simulink model "QAM"  (R2021b)
settings: Solver=VariableStepAuto  StartTime=0.0  StopTime=10.0  RelTol=1e-3
undefined symbols (not defined in the file or in its folder): magnitude
libraries: dspxfrm3 x3, dspsigops x3, commdigbbndam3 x2, commchan3 x1, commrandsrc3 x1
settings Model: Creator=malth  LastModifiedBy=malth

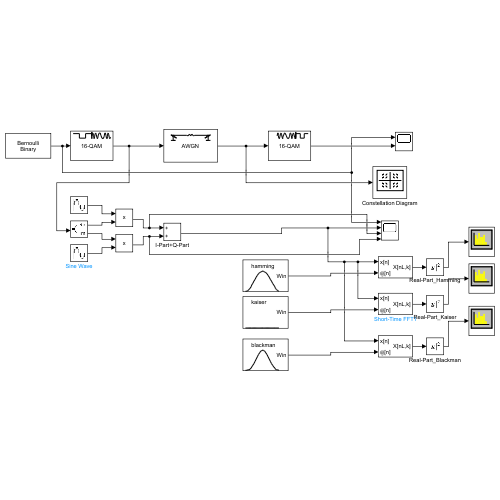
[thumbnail: Simulink's stored preview of the top-level diagram]
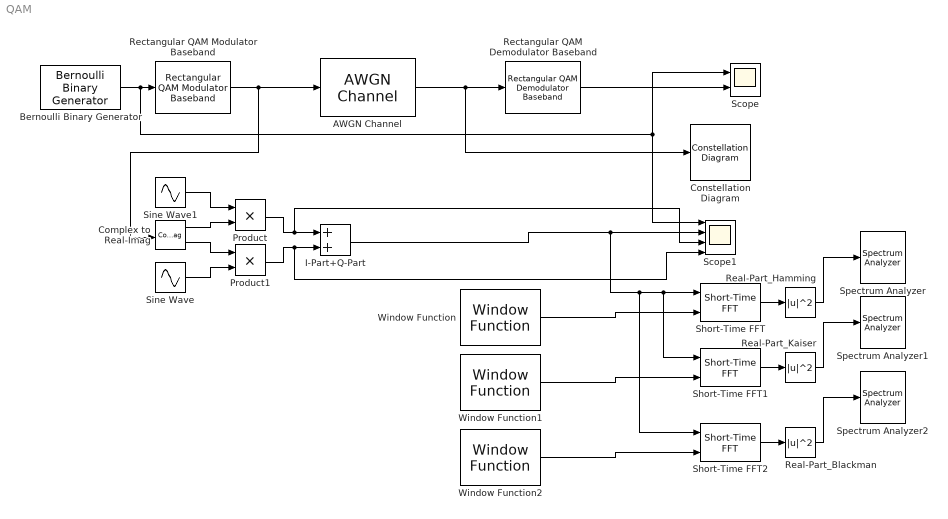
== system QAM ==
  AWGN Channel : commchan3/AWGN Channel  InputProcessing=Columns as channels (frame based)  seed=200  noiseMode="Signal to noise ratio  (Eb/No)"  EbNodB=15  EsNodB=10  SNRdB=10  bitsPerSym=8  Ps=1  Tsym=8  variance=1
  Bernoulli Binary Generator : commrandsrc3/Bernoulli Binary Generator  ProbabilityOfZero=0.5  SeedSource=Auto  Seed=0  SampleTime=1  SamplesPerFrame=8  OutputDataType=boolean  SimulateUsing=Interpreted execution
  Complex to Real-Imag : ComplexToRealImag
  Constellation Diagram : ConstellationDiagram
  I-Part+Q-Part : Sum
  Product : Product
  Product1 : Product
  Real-Part_Blackman : Math  Operator=magnitude^2  OutputSignalType=real  SaturateOnIntegerOverflow=on
  Real-Part_Hamming : Math  Operator=magnitude^2  OutputSignalType=real  SaturateOnIntegerOverflow=on
  Real-Part_Kaiser : Math  Operator=magnitude^2  OutputSignalType=real  SaturateOnIntegerOverflow=on
  Rectangular QAM Demodulator Baseband : commdigbbndam3/Rectangular QAM Demodulator Baseband  M=16  OutType=Bit  DecType=Hard decision  VarSource=Dialog  Variance=1  Dec=Binary  Mapping=[0:15]  PowType=Average Power  MinDist=2  AvgPow=1  PeakPow=1  Ph=0  outDtype1=boolean  outDtype2=Inherit via internal rule  derotateFactorWordLen=16  derotateFactorDataTypeStr=Inherit: Same word length as input  derotateFactorLastDataTypeStr=Inherit: Same word length as input  denormFactorWordLen=16  denormFactorDataTypeStr=Inherit: Same word length as input  denormFactorLastDataTypeStr=Inherit: Same word length as input  prodOutWordLen=32  prodOutOverflowMode=Wrap  prodOutRoundingMode=Floor  prodOutOvFlMode=off  prodOutOvFlModeLastStrValue=off  sumWordLen=32
  Rectangular QAM Modulator Baseband : commdigbbndam3/Rectangular QAM Modulator Baseband  M=16  InType=Bit  Enc=Binary  Mapping=[0:15]  PowType=Average Power  MinDist=2  AvgPow=1  PeakPow=1  Ph=0  outDtype=single  outWordLen=16  outUDDataType=sfix(16)  outFracLenMode=Best precision  outFracLen=15  outDataTypeStr=single  outLastDataTypeStr=single
  Scope : Scope  NumInputPorts=2
  Scope1 : Scope  NumInputPorts=4
  Short-Time FFT : dspxfrm3/Short-Time FFT  W=32  OvLap=4  M=1024
      settings: SourceProductBaseCode=DS
  Short-Time FFT1 : dspxfrm3/Short-Time FFT  W=32  OvLap=4  M=1024
      settings: SourceProductBaseCode=DS
  Short-Time FFT2 : dspxfrm3/Short-Time FFT  W=32  OvLap=4  M=1024
      settings: SourceProductBaseCode=DS
  Sine Wave : Sin  Amplitude=10  Frequency=15079644736.463  Phase=pi/2  SampleTime=0.01
  Sine Wave1 : Sin  Amplitude=10  Frequency=15079644736.463  SampleTime=0.01
  Spectrum Analyzer : SpectrumAnalyzer  IsFrequencyInputMode=1
  Spectrum Analyzer1 : SpectrumAnalyzer  IsFrequencyInputMode=1
  Spectrum Analyzer2 : SpectrumAnalyzer  IsFrequencyInputMode=1
  Window Function : dspsigops/Window Function  winmode=Generate window  wintype=Hamming  sampmode=Discrete  samptime=0.01  N=32  Rs=50  beta=10  winsamp=Periodic  UserWindow=hamming  OptParams=off  UserParams={'symmetric'}  dataType=double  isSigned=on  wordLen=16  udDataType=sfix(16)  fracBitsMode=Best precision  numFracBits=15  roundingMode=Floor  overflowMode=off  numSidelobes=4  sidelobeLevel=-30
      settings: SourceProductBaseCode=DS
  Window Function1 : dspsigops/Window Function  winmode=Generate window  wintype=Kaiser  sampmode=Discrete  samptime=0.01  N=32  Rs=50  beta=2.5  winsamp=Periodic  UserWindow=hamming  OptParams=off  UserParams={'symmetric'}  dataType=double  isSigned=on  wordLen=16  udDataType=sfix(16)  fracBitsMode=Best precision  numFracBits=15  roundingMode=Floor  overflowMode=off  numSidelobes=4  sidelobeLevel=-30
      settings: SourceProductBaseCode=DS
  Window Function2 : dspsigops/Window Function  winmode=Generate window  wintype=Blackman  sampmode=Discrete  samptime=0.01  N=32  Rs=50  beta=10  winsamp=Periodic  UserWindow=hamming  OptParams=off  UserParams={'symmetric'}  dataType=double  isSigned=on  wordLen=16  udDataType=sfix(16)  fracBitsMode=Best precision  numFracBits=15  roundingMode=Floor  overflowMode=off  numSidelobes=4  sidelobeLevel=-30
      settings: SourceProductBaseCode=DS
  wires:
  Rectangular QAM Modulator Baseband/1 -> Complex to Real-Imag/1, AWGN Channel/1
  AWGN Channel/1 -> Constellation Diagram/1, Rectangular QAM Demodulator Baseband/1
  Bernoulli Binary Generator/1 -> Scope1/1, Scope/1, Rectangular QAM Modulator Baseband/1
  Sine Wave/1 -> Product1/2
  Complex to Real-Imag/2 -> Product1/1
  Complex to Real-Imag/1 -> Product/2
  Sine Wave1/1 -> Product/1
  Product/1 -> Scope1/3, I-Part+Q-Part/1
  Product1/1 -> Scope1/4, I-Part+Q-Part/2
  Rectangular QAM Demodulator Baseband/1 -> Scope/2
  Window Function/1 -> Short-Time FFT/2
  I-Part+Q-Part/1 -> Short-Time FFT2/1, Short-Time FFT1/1, Short-Time FFT/1, Scope1/2
  Short-Time FFT/1 -> Real-Part_Hamming/1
  Real-Part_Hamming/1 -> Spectrum Analyzer/1
  Window Function1/1 -> Short-Time FFT1/2
  Short-Time FFT1/1 -> Real-Part_Kaiser/1
  Real-Part_Kaiser/1 -> Spectrum Analyzer1/1
  Window Function2/1 -> Short-Time FFT2/2
  Short-Time FFT2/1 -> Real-Part_Blackman/1
  Real-Part_Blackman/1 -> Spectrum Analyzer2/1
